simulink model "Luenberger_Observer"  (R2022b)
settings: Solver=VariableStepAuto  StartTime=0.0  StopTime=30  RelTol=1e-3
settings Model: Creator=Miakho  LastModifiedBy=Miakho

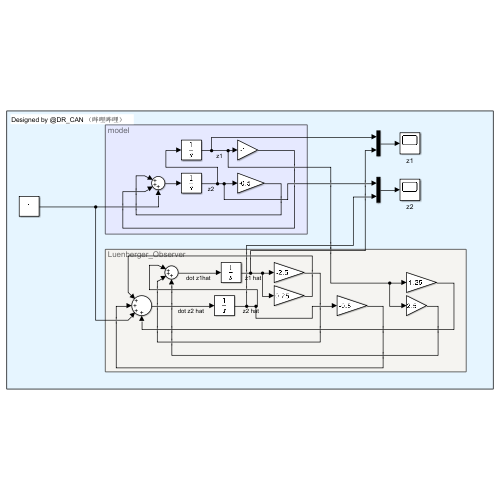
[thumbnail: Simulink's stored preview of the top-level diagram]
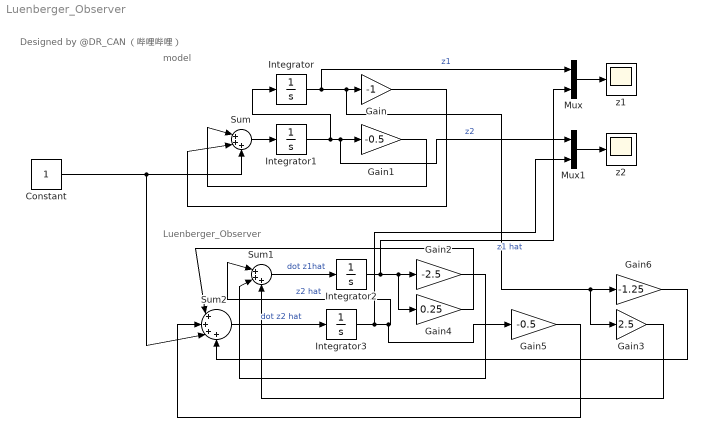
== system Luenberger_Observer ==
  note: Designed by @DR_CAN （哔哩哔哩）
  note: Luenberger_Observer
  note: model
  Constant : Constant
  Gain : Gain  Gain=-1
  Gain1 : Gain  Gain=-0.5
  Gain2 : Gain  Gain=-2.5
  Gain3 : Gain  Gain=2.5
  Gain4 : Gain  Gain=0.25
  Gain5 : Gain  Gain=-0.5
  Gain6 : Gain  Gain=-1.25
  Integrator : Integrator
  Integrator1 : Integrator
  Integrator2 : Integrator  InitialCondition=1
  Integrator3 : Integrator  InitialCondition=1
  Mux : Mux  Inputs=2
  Mux1 : Mux  Inputs=2
  Sum : Sum  Inputs=|+++
  Sum1 : Sum  Inputs=|+++
  Sum2 : Sum  Inputs=|++++
  z1 : Scope
  z2 : Scope
  wires:
  Integrator1/1 -> Mux1/1, Gain1/1, Integrator/1  "z2"
  Integrator/1 -> Mux/1, Gain3/1, Gain6/1, Gain/1  "z1"
  Sum/1 -> Integrator1/1
  Gain/1 -> Sum/2
  Gain1/1 -> Sum/1
  Constant/1 -> Sum2/3, Sum/3
  Integrator2/1 -> Mux/2, Gain4/1, Gain2/1  "z1 hat"
  Sum1/1 -> Integrator2/1  "dot z1hat"
  Integrator3/1 -> Mux1/2, Gain5/1, Sum1/1  "z2 hat"
  Sum2/1 -> Integrator3/1  "dot z2 hat"
  Gain2/1 -> Sum1/2
  Gain3/1 -> Sum1/3
  Gain4/1 -> Sum2/1
  Gain5/1 -> Sum2/2
  Gain6/1 -> Sum2/4
  Mux/1 -> z1/1
  Mux1/1 -> z2/1
